simulink model "amr_mission_supervisor_v05b_readable_low_curve_2026_07_28"  (R2025b)
settings: Solver=FixedStepDiscrete  StartTime=0.0  StopTime=24  FixedStep=0.05  RelTol=1e-3
settings Model: Creator=leeyj  LastModifiedBy=leeyj

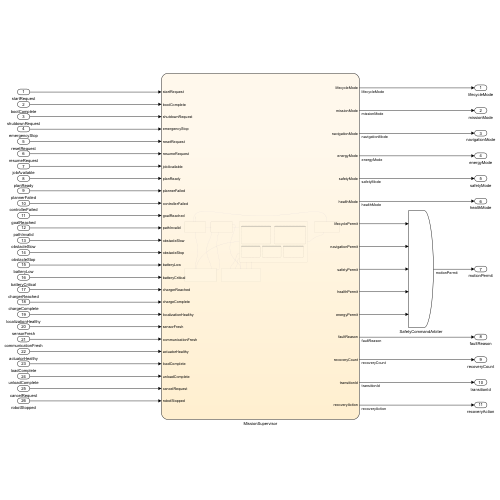
[thumbnail: Simulink's stored preview of the top-level diagram]
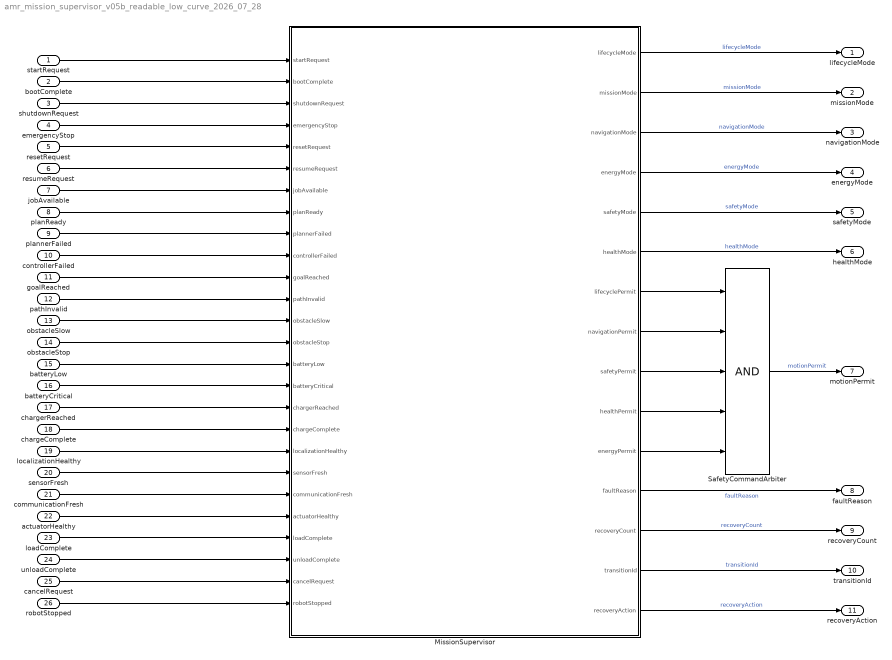
== system amr_mission_supervisor_v05b_readable_low_curve_2026_07_28 ==
  startRequest : Inport
  bootComplete : Inport  Port=2
  shutdownRequest : Inport  Port=3
  emergencyStop : Inport  Port=4
  resetRequest : Inport  Port=5
  resumeRequest : Inport  Port=6
  jobAvailable : Inport  Port=7
  planReady : Inport  Port=8
  plannerFailed : Inport  Port=9
  controllerFailed : Inport  Port=10
  goalReached : Inport  Port=11
  pathInvalid : Inport  Port=12
  obstacleSlow : Inport  Port=13
  obstacleStop : Inport  Port=14
  batteryLow : Inport  Port=15
  batteryCritical : Inport  Port=16
  chargerReached : Inport  Port=17
  chargeComplete : Inport  Port=18
  localizationHealthy : Inport  Port=19
  sensorFresh : Inport  Port=20
  communicationFresh : Inport  Port=21
  actuatorHealthy : Inport  Port=22
  loadComplete : Inport  Port=23
  unloadComplete : Inport  Port=24
  cancelRequest : Inport  Port=25
  robotStopped : Inport  Port=26
  MissionSupervisor : Stateflow chart  TreatAsAtomicUnit=on
  SafetyCommandArbiter : Logic  Inputs=5  IconShape=distinctive
  lifecycleMode : Outport
  missionMode : Outport  Port=2
  navigationMode : Outport  Port=3
  energyMode : Outport  Port=4
  safetyMode : Outport  Port=5
  healthMode : Outport  Port=6
  motionPermit : Outport  Port=7
  faultReason : Outport  Port=8
  recoveryCount : Outport  Port=9
  transitionId : Outport  Port=10
  recoveryAction : Outport  Port=11
  wires:
  SafetyCommandArbiter/1 -> motionPermit/1  "motionPermit"
  startRequest/1 -> MissionSupervisor/1(startRequest)
  bootComplete/1 -> MissionSupervisor/2(bootComplete)
  shutdownRequest/1 -> MissionSupervisor/3(shutdownRequest)
  emergencyStop/1 -> MissionSupervisor/4(emergencyStop)
  resetRequest/1 -> MissionSupervisor/5(resetRequest)
  resumeRequest/1 -> MissionSupervisor/6(resumeRequest)
  jobAvailable/1 -> MissionSupervisor/7(jobAvailable)
  planReady/1 -> MissionSupervisor/8(planReady)
  plannerFailed/1 -> MissionSupervisor/9(plannerFailed)
  controllerFailed/1 -> MissionSupervisor/10(controllerFailed)
  goalReached/1 -> MissionSupervisor/11(goalReached)
  pathInvalid/1 -> MissionSupervisor/12(pathInvalid)
  obstacleSlow/1 -> MissionSupervisor/13(obstacleSlow)
  obstacleStop/1 -> MissionSupervisor/14(obstacleStop)
  batteryLow/1 -> MissionSupervisor/15(batteryLow)
  batteryCritical/1 -> MissionSupervisor/16(batteryCritical)
  chargerReached/1 -> MissionSupervisor/17(chargerReached)
  chargeComplete/1 -> MissionSupervisor/18(chargeComplete)
  localizationHealthy/1 -> MissionSupervisor/19(localizationHealthy)
  sensorFresh/1 -> MissionSupervisor/20(sensorFresh)
  communicationFresh/1 -> MissionSupervisor/21(communicationFresh)
  actuatorHealthy/1 -> MissionSupervisor/22(actuatorHealthy)
  loadComplete/1 -> MissionSupervisor/23(loadComplete)
  unloadComplete/1 -> MissionSupervisor/24(unloadComplete)
  cancelRequest/1 -> MissionSupervisor/25(cancelRequest)
  robotStopped/1 -> MissionSupervisor/26(robotStopped)
  MissionSupervisor/1(lifecycleMode) -> lifecycleMode/1  "lifecycleMode"
  MissionSupervisor/2(missionMode) -> missionMode/1  "missionMode"
  MissionSupervisor/3(navigationMode) -> navigationMode/1  "navigationMode"
  MissionSupervisor/4(energyMode) -> energyMode/1  "energyMode"
  MissionSupervisor/5(safetyMode) -> safetyMode/1  "safetyMode"
  MissionSupervisor/6(healthMode) -> healthMode/1  "healthMode"
  MissionSupervisor/7(lifecyclePermit) -> SafetyCommandArbiter/1
  MissionSupervisor/8(navigationPermit) -> SafetyCommandArbiter/2
  MissionSupervisor/9(safetyPermit) -> SafetyCommandArbiter/3
  MissionSupervisor/10(healthPermit) -> SafetyCommandArbiter/4
  MissionSupervisor/11(energyPermit) -> SafetyCommandArbiter/5
  MissionSupervisor/12(faultReason) -> faultReason/1  "faultReason"
  MissionSupervisor/13(recoveryCount) -> recoveryCount/1  "recoveryCount"
  MissionSupervisor/14(transitionId) -> transitionId/1  "transitionId"
  MissionSupervisor/15(recoveryAction) -> recoveryAction/1  "recoveryAction"

== stateflow chart amr_mission_supervisor_v05b_readable_low_curve_2026_07_28/MissionSupervisor ==
  state PowerOff
    en:
    lifecycleMode = amr.supervision.LifecycleMode.PowerOff;
    missionMode = amr.supervision.MissionMode.Idle;
    navigationMode = amr.supervision.NavigationMode.NavIdle;
    energyMode = amr.supervision.EnergyMode.Normal;
    safetyMode = amr.supervision.SafetyMode.Clear;
    healthMode = amr.supervision.HealthMode.Healthy;
    lifecyclePermit = false;
    navigationPermit = false;
    safetyPermit = false;
    healthPermit = false;
    energyPermit = false;
    faultReason = amr.supervision.FaultReason.None;
    recoveryCountLocal = uint8(0);
    recoveryCount = uint8(0);
    transitionId = uint16(100);
    recoveryAction = amr.supervision.RecoveryAction.None;
  state Boot
    en:
    lifecycleMode = amr.supervision.LifecycleMode.Boot;
    missionMode = amr.supervision.MissionMode.Idle;
    navigationMode = amr.supervision.NavigationMode.NavIdle;
    energyMode = amr.supervision.EnergyMode.Normal;
    safetyMode = amr.supervision.SafetyMode.Clear;
    healthMode = amr.supervision.HealthMode.Healthy;
    lifecyclePermit = false;
    navigationPermit = false;
    safetyPermit = false;
    healthPermit = false;
    energyPermit = false;
    faultReason = amr.supervision.FaultReason.None;
    recoveryCountLocal = uint8(0);
    recoveryCount = uint8(0);
    transitionId = uint16(101);
    recoveryAction = amr.supervision.RecoveryAction.None;
  state Operational
    en:
    lifecycleMode = amr.supervision.LifecycleMode.Operational;
    lifecyclePermit = true;
    transitionId = uint16(102);
    state MissionRegion [parallel]
      settings: executionOrder=1
      state Idle
        en:
        missionMode = amr.supervision.MissionMode.Idle;
      state ValidateJob
        en:
        missionMode = amr.supervision.MissionMode.ValidateJob;
      state NavigatePickup
        en:
        missionMode = amr.supervision.MissionMode.NavigatePickup;
      state Loading
        en:
        missionMode = amr.supervision.MissionMode.Loading;
      state NavigateDropoff
        en:
        missionMode = amr.supervision.MissionMode.NavigateDropoff;
      state Unloading
        en:
        missionMode = amr.supervision.MissionMode.Unloading;
      state ReturnHome
        en:
        missionMode = amr.supervision.MissionMode.ReturnHome;
      state Completed
        en:
        missionMode = amr.supervision.MissionMode.Completed;
      state Aborting
        en:
        missionMode = amr.supervision.MissionMode.Aborting;
      Aborting -> Idle : after(0.2,sec)
      NavigateDropoff -> Aborting [order 2] : [cancelRequest]
      ValidateJob -> Aborting [order 2] : after(1,sec)
      Unloading -> Aborting [order 1] : [cancelRequest]
      NavigatePickup -> Aborting [order 2] : [cancelRequest]
      Loading -> Aborting [order 1] : [cancelRequest]
      Unloading -> Aborting [order 3] : after(3,sec)
      Loading -> Aborting [order 3] : after(3,sec)
      ReturnHome -> Aborting [order 2] : [cancelRequest]
      Completed -> Idle : after(0.1,sec)
      (default) -> Idle
      Idle -> ValidateJob : [jobAvailable]
      ValidateJob -> NavigatePickup [order 1] : [jobAvailable]
      NavigatePickup -> Loading [order 1] : [goalReached]
      Loading -> NavigateDropoff [order 2] : [loadComplete]
      NavigateDropoff -> Unloading [order 1] : [goalReached]
      Unloading -> ReturnHome [order 2] : [unloadComplete]
      ReturnHome -> Completed [order 1] : [goalReached]
    state NavigationRegion [parallel]
      settings: executionOrder=4
      state NavIdle
        en:
        navigationMode = amr.supervision.NavigationMode.NavIdle;
        navigationPermit = false;
        recoveryAction = amr.supervision.RecoveryAction.None;
      state Planning
        en:
        navigationMode = amr.supervision.NavigationMode.Planning;
        navigationPermit = false;
        recoveryAction = amr.supervision.RecoveryAction.Replan;
      state Tracking
        en:
        navigationMode = amr.supervision.NavigationMode.Tracking;
        navigationPermit = true;
        recoveryAction = amr.supervision.RecoveryAction.None;
      state Recovery
        en:
        navigationMode = amr.supervision.NavigationMode.Recovery;
        navigationPermit = false;
        recoveryCountLocal = recoveryCountLocal + uint8(1);
        recoveryCount = recoveryCountLocal;
        if recoveryCountLocal == uint8(1)
        recoveryAction = amr.supervision.RecoveryAction.ClearLocalMap;
        else
        recoveryAction = amr.supervision.RecoveryAction.RequestAssistance;
        end
      state NavFailed
        en:
        navigationMode = amr.supervision.NavigationMode.NavFailed;
        navigationPermit = false;
        recoveryAction = amr.supervision.RecoveryAction.AbortMission;
      state Replanning
        en:
        navigationMode = amr.supervision.NavigationMode.Replanning;
        navigationPermit = false;
        recoveryAction = amr.supervision.RecoveryAction.Replan;
      Tracking -> Replanning [order 1] : [pathInvalid]
      Replanning -> Recovery [order 3] : after(3,sec)
      Replanning -> Recovery [order 2] : [plannerFailed]
      Tracking -> NavIdle [order 3] : [goalReached]{recoveryCountLocal = uint8(0); recoveryCount = uint8(0);}
      (default) -> NavIdle
      Replanning -> Tracking [order 1] : [planReady && ~plannerFailed]
      NavIdle -> Planning : [missionMode == amr.supervision.MissionMode.NavigatePickup || missionMode == amr.supervision.MissionMode.NavigateDropoff || missionMode == amr.supervision.MissionMode.ReturnHome]
      Planning -> Tracking [order 1] : [planReady && ~plannerFailed]
      Recovery -> Planning [order 2] : [after(0.5,sec) && recoveryCountLocal < uint8(2)]
      Tracking -> Recovery [order 2] : [controllerFailed]
      Recovery -> Planning [order 1] : [resumeRequest && recoveryCountLocal <= uint8(2)]
      Planning -> Recovery [order 2] : [plannerFailed]
      Planning -> Recovery [order 3] : after(3,sec)
      Recovery -> NavFailed [order 3] : after(2,sec)
    state SafetyRegion [parallel]
      settings: executionOrder=2
      state SafetyClear
        en:
        safetyMode = amr.supervision.SafetyMode.Clear;
        safetyPermit = true;
      state Slowdown
        en:
        safetyMode = amr.supervision.SafetyMode.Slowdown;
        safetyPermit = true;
      state ProtectiveStop
        en:
        safetyMode = amr.supervision.SafetyMode.ProtectiveStop;
        safetyPermit = false;
      ProtectiveStop -> SafetyClear : [resumeRequest && ~obstacleStop && sensorFresh && communicationFresh && localizationHealthy]
      (default) -> SafetyClear
      Slowdown -> SafetyClear [order 2] : [~obstacleSlow && ~obstacleStop]
      SafetyClear -> ProtectiveStop [order 1] : [obstacleStop || ~sensorFresh || ~communicationFresh || ~localizationHealthy]
      SafetyClear -> Slowdown [order 2] : [obstacleSlow]
      Slowdown -> ProtectiveStop [order 1] : [obstacleStop || ~sensorFresh || ~communicationFresh || ~localizationHealthy]
    state HealthRegion [parallel]
      settings: executionOrder=3
      state Healthy
        en:
        healthMode = amr.supervision.HealthMode.Healthy;
        healthPermit = true;
      state Degraded
        en:
        healthMode = amr.supervision.HealthMode.Degraded;
        healthPermit = true;
      state FaultRequest
        en:
        healthMode = amr.supervision.HealthMode.FaultRequest;
        healthPermit = false;
      (default) -> Healthy
      Degraded -> Healthy [order 2] : [sensorFresh && communicationFresh && localizationHealthy && actuatorHealthy]
      Healthy -> FaultRequest [order 1] : [~actuatorHealthy]
      Degraded -> FaultRequest [order 3] : after(3,sec)
      Healthy -> Degraded [order 2] : [~sensorFresh || ~communicationFresh || ~localizationHealthy]
      Degraded -> FaultRequest [order 1] : [~actuatorHealthy]
    state EnergyRegion [parallel]
      settings: executionOrder=5
      state EnergyNormal
        en:
        energyMode = amr.supervision.EnergyMode.Normal;
        energyPermit = true;
      state EnergyLow
        en:
        energyMode = amr.supervision.EnergyMode.Low;
        energyPermit = true;
      state EnergyCritical
        en:
        energyMode = amr.supervision.EnergyMode.Critical;
        energyPermit = false;
      state GoToCharger
        en:
        energyMode = amr.supervision.EnergyMode.GoToCharger;
        energyPermit = true;
      state Charging
        en:
        energyMode = amr.supervision.EnergyMode.Charging;
        energyPermit = false;
      EnergyCritical -> Charging [order 1] : [chargerReached]
      GoToCharger -> Charging : [chargerReached]
      (default) -> EnergyNormal
      EnergyLow -> EnergyNormal [order 2] : [~batteryLow]
      EnergyNormal -> EnergyLow : [batteryLow]
      EnergyLow -> EnergyCritical [order 1] : [batteryCritical]
      EnergyCritical -> GoToCharger [order 2] : after(0.1,sec)
      Charging -> EnergyNormal : [chargeComplete]
  state ControlledShutdown
    en:
    lifecycleMode = amr.supervision.LifecycleMode.ControlledShutdown;
    missionMode = amr.supervision.MissionMode.Idle;
    navigationMode = amr.supervision.NavigationMode.NavIdle;
    lifecyclePermit = false;
    navigationPermit = false;
    safetyPermit = false;
    healthPermit = false;
    energyPermit = false;
    transitionId = uint16(103);
    recoveryAction = amr.supervision.RecoveryAction.None;
  state EmergencyStopLatched
    en:
    lifecycleMode = amr.supervision.LifecycleMode.EmergencyStopLatched;
    missionMode = amr.supervision.MissionMode.Suspended;
    navigationMode = amr.supervision.NavigationMode.NavIdle;
    safetyMode = amr.supervision.SafetyMode.ProtectiveStop;
    healthMode = amr.supervision.HealthMode.Degraded;
    lifecyclePermit = false;
    navigationPermit = false;
    safetyPermit = false;
    healthPermit = false;
    energyPermit = false;
    faultReason = amr.supervision.FaultReason.EmergencyStop;
    transitionId = uint16(105);
    recoveryAction = amr.supervision.RecoveryAction.None;
  state FaultLatched
    en:
    lifecycleMode = amr.supervision.LifecycleMode.FaultLatched;
    missionMode = amr.supervision.MissionMode.Aborting;
    navigationMode = amr.supervision.NavigationMode.NavFailed;
    safetyMode = amr.supervision.SafetyMode.ProtectiveStop;
    healthMode = amr.supervision.HealthMode.FaultRequest;
    lifecyclePermit = false;
    navigationPermit = false;
    safetyPermit = false;
    healthPermit = false;
    energyPermit = false;
    transitionId = uint16(104);
    recoveryAction = amr.supervision.RecoveryAction.AbortMission;
  ControlledShutdown -> PowerOff : after(1,sec)
  (default) -> PowerOff
  PowerOff -> Boot [order 2] : [startRequest && ~emergencyStop]
  Boot -> Operational [order 2] : [bootComplete && actuatorHealthy && sensorFresh && communicationFresh && localizationHealthy]
  PowerOff -> EmergencyStopLatched [order 1] : [emergencyStop]
  Boot -> EmergencyStopLatched [order 1] : [emergencyStop]
  EmergencyStopLatched -> Boot : [resetRequest && ~emergencyStop && robotStopped && actuatorHealthy && sensorFresh && communicationFresh && localizationHealthy]
  FaultLatched -> Boot : [resetRequest && robotStopped && actuatorHealthy && sensorFresh && communicationFresh && localizationHealthy]
  Operational -> ControlledShutdown [order 7] : [shutdownRequest]
  Operational -> EmergencyStopLatched [order 1] : [emergencyStop]
  Operational -> FaultLatched [order 2] : [~actuatorHealthy]{faultReason = amr.supervision.FaultReason.DriveFault;}
  Operational -> FaultLatched [order 3] : [navigationMode == amr.supervision.NavigationMode.NavFailed]{faultReason = amr.supervision.FaultReason.RecoveryExhausted;}
  Operational -> FaultLatched [order 4] : [healthMode == amr.supervision.HealthMode.FaultRequest && ~communicationFresh]{faultReason = amr.supervision.FaultReason.CommunicationLost;}
  Operational -> FaultLatched [order 6] : [healthMode == amr.supervision.HealthMode.FaultRequest && communicationFresh && localizationHealthy]{faultReason = amr.supervision.FaultReason.SafetySensorStale;}
  Operational -> FaultLatched [order 5] : [healthMode == amr.supervision.HealthMode.FaultRequest && communicationFresh && ~localizationHealthy]{faultReason = amr.supervision.FaultReason.LocalizationInvalid;}
  data: startRequest input boolean; bootComplete input boolean; shutdownRequest input boolean; emergencyStop input boolean; resetRequest input boolean; resumeRequest input boolean; jobAvailable input boolean; planReady input boolean; plannerFailed input boolean; controllerFailed input boolean; goalReached input boolean; pathInvalid input boolean; obstacleSlow input boolean; obstacleStop input boolean; batteryLow input boolean; batteryCritical input boolean; chargerReached input boolean; chargeComplete input boolean; localizationHealthy input boolean; sensorFresh input boolean; communicationFresh input boolean; actuatorHealthy input boolean; loadComplete input boolean; unloadComplete input boolean; cancelRequest input boolean; robotStopped input boolean; lifecycleMode output Enum: amr.supervision.LifecycleMode; missionMode output Enum: amr.supervision.MissionMode; navigationMode output Enum: amr.supervision.NavigationMode; energyMode output Enum: amr.supervision.EnergyMode; safetyMode output Enum: amr.supervision.SafetyMode; healthMode output Enum: amr.supervision.HealthMode; lifecyclePermit output boolean; navigationPermit output boolean; safetyPermit output boolean; healthPermit output boolean; energyPermit output boolean; faultReason output Enum: amr.supervision.FaultReason; recoveryCount output uint8; transitionId output uint16; recoveryAction output Enum: amr.supervision.RecoveryAction; recoveryCountLocal local uint8
